simulink model "speed_modelo_motor_frenado"  (R2022b)
settings: Solver=VariableStepAuto  StartTime=0.0  StopTime=10  FixedStep=0.01  MaxStep=0.00005  RelTol=1e-3
values from neighbouring files (symbols this model uses):
  airgap_drag = [8 13 18 23]    [datos_modelo.mat]
  Force_drag = [-0.0263599613947 43.4567385798 79.8814932025 112.890713456 143.193346103 171.145741633 196.959308063 220.848934943 -0.0285293042528 24.6775545387 45.2474492116 63.9699604043 ... (32 elements, 8x4)]    [datos_modelo.mat]
  frecuencia = (3:3:48)    [carga_datos_motor_simple.m]    (also in datos_modelo.mat = [3 6 9 12 15 18 21 24 27 30 33 36 ... (16 elements, 1x16)])
  frecuencia_freno = -48:3:-3    [carga_datos_frenado_v3.m]    (also in carga_datos_frenado_v4.m; datos_modelo.mat = [-48 -45 -42 -39 -36 -33 -30 -27 -24 -21 -18 -15 ... (16 ele)
  FuerzaX_acel = []    [carga_datos_motor_simple.m]    (also in datos_modelo.mat = [0.156686825585 1.1015935563 2.01038201102 2.86930542934 3.6)
  FuerzaX_freno = []    [carga_datos_frenado_v3.m]    (also in datos_modelo.mat = [153.020892613 -180.239809195 -245.613894698 -262.756397176 )
  FuerzaY_acel = []    [carga_datos_motor_simple.m]    (also in datos_modelo.mat = [16.7719587108 16.6669307493 16.4360183454 16.0997979621 15.)
  Ipeak = (10:10:100)    [carga_datos_fuerza_laterales.m]    (also in carga_datos_motor_simple.m; datos_modelo.mat = [10 20 30 40 50 60 70 80 90 100])
  L = [0.00288301128086 0.00287460594326 0.00286413458194 0.00286292567045 0.00283652697085 0.00271657977235 0.0024764202896 0.0021234760901 0.00287319201871 0.00287259972172 0.0028679034407 0.0028580918991 ... (1408 elements, 8x11x16)]    [datos_modelo.mat]
  mass = 200    [datos_modelo.mat]
  p1 = 1.3    [datos_modelo.mat]
  p2 = 8.4    [datos_modelo.mat]
  pole_length = 0.114    [datos_modelo.mat]
  r = 0.384    [datos_modelo.mat]
  slip = (1:-0.1:0)    [carga_datos_motor_simple.m]    (also in datos_modelo.mat = [0 0.1 0.2 0.3 0.4 0.5 0.6 0.7 0.8 0.9 1])
  vel_drag = [0 5 10 15 20 25 30 35]    [datos_modelo.mat]
  vel_motor_freno = vel_motor_freno*3.6    [carga_datos_frenado_v3.m]    (also in datos_modelo.mat = [4.9248 9.8496 14.7744 19.6992 24.624 29.5488 34.4736 39.398)
libraries: slpidlib x2, eePowerMeasurement x1
settings Model: Creator=mique  LastModifiedBy=mique
settings SolverCC: ZeroCrossAlgorithm=Adaptive
settings DebuggingCC: IgnoredZcDiagnostic=none

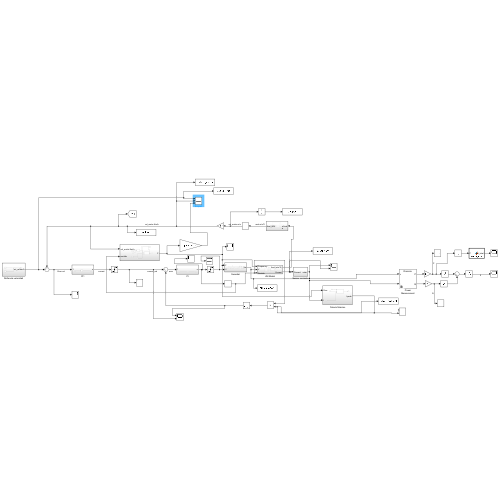
[thumbnail: Simulink's stored preview of the top-level diagram]
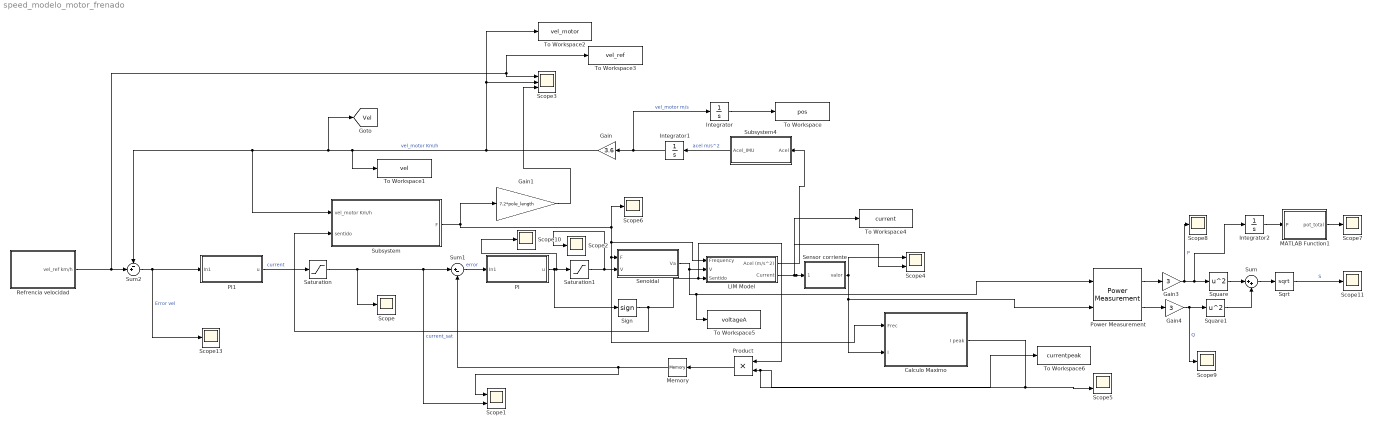
== system speed_modelo_motor_frenado ==
  Calculo Maximo : Subsystem
  Gain : Gain  Gain=3.6
  Gain1 : Gain  Gain=7.2*pole_length
  Gain3 : Gain  Gain=3
  Gain4 : Gain  Gain=3
  Integrator : Integrator
  Integrator1 : Integrator
  Integrator2 : Integrator
  LIM Model : Subsystem
  MATLAB Function1 : MATLAB Function  TreatAsAtomicUnit=on
  Memory : Memory
  PI : Subsystem
  PI1 : Subsystem
  Power Measurement : eePowerMeasurement/Power Measurement  LabelModeActiveChoice=Discrete  F=8  K=[0 1 2 3 4 5 6 7 8 9 10 11]  Ts=0.0002
  Product : Product
  Refrencia velocidad : Subsystem
  Saturation : Saturate  UpperLimit=100  LowerLimit=-100
  Saturation1 : Saturate  UpperLimit=200  LowerLimit=-200
  Scope{,2,6..11,13} (9 alike) : Scope
  Scope1 : Scope  NumInputPorts=2
  Scope3 : Scope  NumInputPorts=3
  Scope4 : Scope  NumInputPorts=2
  Scope5 : Scope  NumInputPorts=2
  Senoidal : Subsystem
  Sensor corriente : Subsystem
  Sign : Signum
  Sqrt : Sqrt
  Square : Math  Operator=square
  Square1 : Math  Operator=square
  Subsystem : Subsystem
  Subsystem4 : Subsystem
  Sum : Sum  Inputs=|++
  Sum1 : Sum  Inputs=|+-
  Sum2 : Sum  Inputs=-+|
  To Workspace : ToWorkspace  VariableName=pos  SampleTime=-1
  To Workspace1 : ToWorkspace  VariableName=vel  SampleTime=-1
  To Workspace2 : ToWorkspace  VariableName=vel_motor  SampleTime=-1
  To Workspace3 : ToWorkspace  VariableName=vel_ref  SampleTime=-1
  To Workspace4 : ToWorkspace  VariableName=current  SampleTime=-1
  To Workspace5 : ToWorkspace  VariableName=voltageA  SaveFormat=Timeseries  SampleTime=-1
  To Workspace6 : ToWorkspace  VariableName=currentpeak  SampleTime=-1
  tag scope: Vel=global
  wires:
  Integrator1/1 -> Integrator/1, Gain/1  "vel_motor m/s"
  Gain/1 -> To Workspace2/1, Scope3/2, To Workspace1/1, [Vel], Subsystem/1(vel_motor Km/h), Sum2/1  "vel_motor Km/h"
  LIM Model/1(Acel (m/s^2)) -> Subsystem4/1(Acel)
  Integrator/1 -> To Workspace/1
  Sum1/1 -> PI/1(In1)  "error"
  Sum2/1 -> PI1/1(In1), Scope13/1  "Error vel"
  Refrencia velocidad/1(vel_ref km/h) -> To Workspace3/1, Scope3/1, Sum2/2
  PI1/1(u) -> Saturation/1  "current"
  Gain1/1 -> Scope3/3
  Saturation/1 -> Scope/1, Scope1/2, Sum1/1  "current_sat"
  Subsystem4/1(Acel_IMU) -> Integrator1/1  "acel m/s^2"
  Senoidal/1(Va) -> To Workspace5/1, Power Measurement/1, LIM Model/2("V ")
  Power Measurement/1 -> Gain3/1
  Gain3/1 -> Integrator2/1, Square/1, Scope8/1  "P"
  Power Measurement/2 -> Gain4/1
  Gain4/1 -> Scope9/1, Square1/1  "Q"
  Square/1 -> Sum/1
  Square1/1 -> Sum/2
  Sum/1 -> Sqrt/1
  Sqrt/1 -> Scope11/1  "S"
  Sign/1 -> Subsystem/2(sentido), Product/1, LIM Model/3(Sentido)
  Product/1 -> Memory/1
  Memory/1 -> Scope1/1, Sum1/2
  Sensor corriente/1(valor) -> Scope4/1, Calculo Maximo/2(I), Power Measurement/2
  PI/1(u) -> Sign/1, Scope10/1, Saturation1/1
  Saturation1/1 -> Scope2/1, Senoidal/2(V)
  Integrator2/1 -> MATLAB Function1/1(P)
  MATLAB Function1/1(pot_total) -> Scope7/1
  Subsystem/1(F) -> Gain1/1, Scope6/1, Calculo Maximo/1(Frec), Senoidal/1(F), LIM Model/1(Frequency)
  Calculo Maximo/1(I peak) -> To Workspace6/1, Product/2, Scope5/2
  LIM Model/2(Current) -> Scope4/2, To Workspace4/1, Sensor corriente/1(Current)

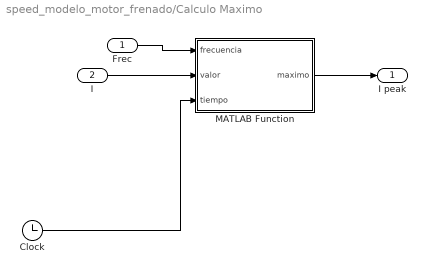
== system speed_modelo_motor_frenado/Calculo Maximo ==
  Frec : Inport
  I : Inport  Port=2
  Clock : Clock
  MATLAB Function : MATLAB Function  TreatAsAtomicUnit=on
  I peak : Outport
  wires:
  Frec/1 -> MATLAB Function/1(frecuencia)
  I/1 -> MATLAB Function/2(valor)
  MATLAB Function/1(maximo) -> I peak/1
  Clock/1 -> MATLAB Function/3(tiempo)

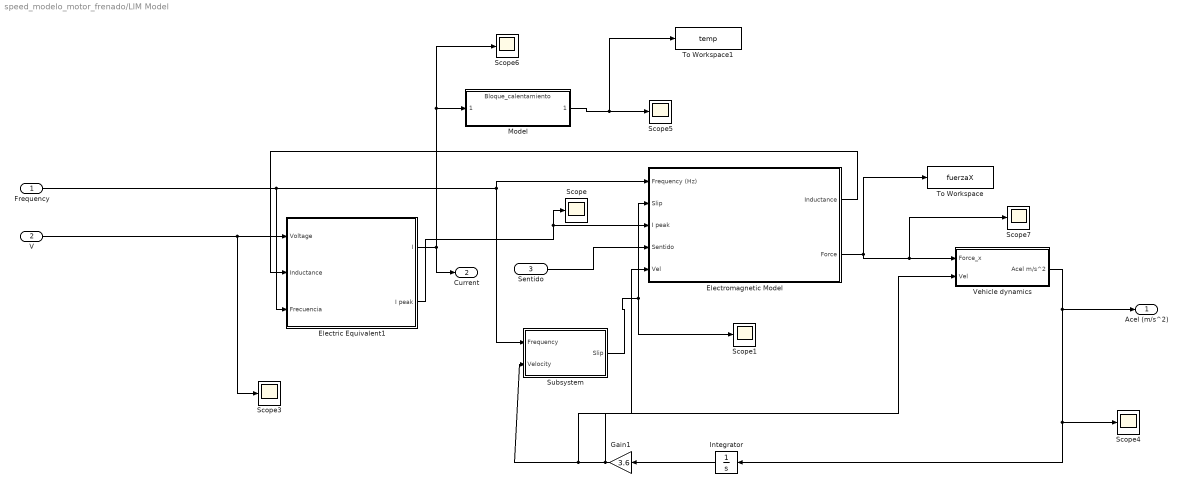
== system speed_modelo_motor_frenado/LIM Model ==
  Frequency : Inport
  "V " : Inport  Port=2
  Sentido : Inport  Port=3
  Electric Equivalent1 : Subsystem
  Electromagnetic Model : Subsystem
  Gain1 : Gain  Gain=3.6
  Integrator : Integrator
  Model : ModelReference  ModelNameDialog=Bloque_calentamiento.slx  SimulationMode=Normal  ModelReferenceVersion=3.8
  Scope{,1,3..7} (7 alike) : Scope
  Subsystem : Subsystem
  To Workspace : ToWorkspace  VariableName=fuerzaX  SampleTime=-1
  To Workspace1 : ToWorkspace  VariableName=temp  SampleTime=-1
  Vehicle dynamics : Subsystem
  Acel (m/s^2) : Outport
  Current : Outport  Port=2
  wires:
  Vehicle dynamics/1(Acel m/s^2) -> Integrator/1, Scope4/1, Acel (m/s^2)/1
  Electric Equivalent1/2(I peak) -> Scope/1, Electromagnetic Model/3(I peak)
  Electromagnetic Model/1(Inductance) -> Electric Equivalent1/2(Inductance)
  Frequency/1 -> Electric Equivalent1/3(Frecuencia), Subsystem/1(Frequency), Electromagnetic Model/1(Frequency (Hz))
  Integrator/1 -> Gain1/1
  "V "/1 -> Scope3/1, Electric Equivalent1/1(Voltage)
  Model/1 -> To Workspace1/1, Scope5/1
  Electric Equivalent1/1("I ") -> Current/1, Scope6/1, Model/1
  Sentido/1 -> Electromagnetic Model/4(Sentido)
  Subsystem/1(Slip) -> Scope1/1, Electromagnetic Model/2(Slip)
  Gain1/1 -> Vehicle dynamics/2(Vel), Electromagnetic Model/5(Vel), Subsystem/2(Velocity)
  Electromagnetic Model/2(Force) -> To Workspace/1, Scope7/1, Vehicle dynamics/1(Force_x)

== system speed_modelo_motor_frenado/PI ==
  note: Parametros obtenidos con el PID tuner
  In1 : Inport
  Discrete PID Controller1 : slpidlib/PID Controller  Controller=PI  Form=Parallel  TimeDomain=Discrete-time  UseExternalTs=off  SampleTime=0.0002  IntegratorMethod=Forward Euler  FilterMethod=Forward Euler  ControllerParametersSource=internal  P=0.3  I=5  UseKiTs=off  D=0.5  N=10  UseFilter=on  TunerSelectOption=Transfer Function Based (PID Tuner App)  InitialConditionSource=internal  InitialConditionForIntegrator=0  InitialConditionForFilter=0  DifferentiatorICPrevScaledInput=0  ExternalReset=none  TrackingMode=off  Kt=1  LimitOutput=off  SatLimitsSource=internal  UpperSaturationLimit=100  LowerSaturationLimit=-inf  LinearizeAsGain=off  AntiWindupMode=back-calculation  Kb=1  LimitIntegrator=off  UpperIntegratorSaturationLimit=15  LowerIntegratorSaturationLimit=-15  POutMin=[]  POutMax=[]  IOutMin=[]  IOutMax=[]  DOutMin=[]  DOutMax=[]  NOutMin=[]  NOutMax=[]  SumOutMin=[]  SumOutMax=[]  SaturationOutMin=[]  SaturationOutMax=[]  PParamMin=[]  PParamMax=[]  IParamMin=[]  IParamMax=[]  DParamMin=[]  DParamMax=[]  NParamMin=[]  NParamMax=[]  KbParamMin=[]  KbParamMax=[]  KtParamMin=[]  KtParamMax=[]  KbOutMin=[]  KbOutMax=[]  KtOutMin=[]  KtOutMax=[]  IntegratorOutMin=[]  IntegratorOutMax=[]  FilterOutMin=[]  FilterOutMax=[]  SumI1OutMin=[]  SumI1OutMax=[]  SumI2OutMin=[]  SumI2OutMax=[]  SumI3OutMin=[]  SumI3OutMax=[]  SumI4OutMin=[]  SumI4OutMax=[]  SumDOutMin=[]  SumDOutMax=[]  DifferentiatorOutMin=[]  DifferentiatorOutMax=[]  FilterDiffOutCoefMin=[]  FilterDiffOutCoefMax=[]  ReciprocalOutMin=[]  ReciprocalOutMax=[]  SumDenOutMin=[]  SumDenOutMax=[]  SumNumOutMin=[]  SumNumOutMax=[]  DivideOutMin=[]  DivideOutMax=[]  UdiffTsProdOutMin=[]  UdiffTsProdOutMax=[]  NTsProdOutMin=[]  NTsProdOutMax=[]  UintegralTsProdOutMin=[]  UintegralTsProdOutMax=[]  UngainTsProdOutMin=[]  UngainTsProdOutMax=[]  ClampingZeroOutDataTypeStr=Inherit: Inherit via back propagation  ClampingZeroOutMin=[]  ClampingZeroOutMax=[]  FilterDenConstantOutDataTypeStr=Inherit: Inherit via back propagation  FilterDenConstantOutMin=[]  FilterDenConstantOutMax=[]  PCopyOutDataTypeStr=Inherit: Inherit via back propagation  PCopyOutMin=[]  PCopyOutMax=[]  NCopyOutDataTypeStr=Inherit: Inherit via back propagation  NCopyOutMin=[]  NCopyOutMax=[]  IntegratorContinuousStateAttributes=''  IntegratorStateMustResolveToSignalObject=off  IntegratorRTWStateStorageClass=Auto  FilterContinuousStateAttributes=''  FilterStateMustResolveToSignalObject=off  FilterRTWStateStorageClass=Auto  ParallelPVariant=InternalParameters  IdealPVariant=Disabled  IVariant=InternalParameters  DVariant=Disabled  IntegratorVariant=Discrete  SatVariant=Disabled  AWVariant=Passthrough  PCopyVariant=Disabled  TRVariant=Disabled  FdbkBlocksVariant=Forward  IdealPFdbkVariant=Disabled  SatFdbkVariant=Disabled  DerivativeFilterVariant=Disabled  NVariant=Disabled  NCopyVariant=Disabled_SignalSpec  FilterICVariant=Disabled  IntegratorICVariant=InternalICs  ExternalResetVariant=Disabled  TRSumVariant=Passthrough  SumFdbkVariant=Disabled  SumVariant=Sum_PI  TsampFilterVariant=InternalTs  TsampNgainVariant=Passthrough  TsampIntegralVariant=Passthrough  ExternalSaturationOutDataTypeStr=Inherit: Same as second input
      settings: LibrarySourceBlock=simulink/Discrete/Discrete PID Controller
  u : Outport
  wires:
  In1/1 -> Discrete PID Controller1/1
  Discrete PID Controller1/1 -> u/1

== system speed_modelo_motor_frenado/PI1 ==
  note: Parametros obtenidos con el PID tuner
  In1 : Inport
  Discrete PID Controller1 : slpidlib/PID Controller  Controller=PI  Form=Parallel  TimeDomain=Discrete-time  UseExternalTs=off  SampleTime=0.001  IntegratorMethod=Forward Euler  FilterMethod=Forward Euler  ControllerParametersSource=internal  P=300  I=25  UseKiTs=off  D=0.2  N=10  UseFilter=on  TunerSelectOption=Transfer Function Based (PID Tuner App)  InitialConditionSource=internal  InitialConditionForIntegrator=0  InitialConditionForFilter=0  DifferentiatorICPrevScaledInput=0  ExternalReset=none  TrackingMode=off  Kt=1  LimitOutput=off  SatLimitsSource=internal  UpperSaturationLimit=100  LowerSaturationLimit=-100  LinearizeAsGain=off  AntiWindupMode=clamping  Kb=0.1  LimitIntegrator=on  UpperIntegratorSaturationLimit=15  LowerIntegratorSaturationLimit=-15  POutMin=[]  POutMax=[]  IOutMin=[]  IOutMax=[]  DOutMin=[]  DOutMax=[]  NOutMin=[]  NOutMax=[]  SumOutMin=[]  SumOutMax=[]  SaturationOutMin=[]  SaturationOutMax=[]  PParamMin=[]  PParamMax=[]  IParamMin=[]  IParamMax=[]  DParamMin=[]  DParamMax=[]  NParamMin=[]  NParamMax=[]  KbParamMin=[]  KbParamMax=[]  KtParamMin=[]  KtParamMax=[]  KbOutMin=[]  KbOutMax=[]  KtOutMin=[]  KtOutMax=[]  IntegratorOutMin=[]  IntegratorOutMax=[]  FilterOutMin=[]  FilterOutMax=[]  SumI1OutMin=[]  SumI1OutMax=[]  SumI2OutMin=[]  SumI2OutMax=[]  SumI3OutMin=[]  SumI3OutMax=[]  SumI4OutMin=[]  SumI4OutMax=[]  SumDOutMin=[]  SumDOutMax=[]  DifferentiatorOutMin=[]  DifferentiatorOutMax=[]  FilterDiffOutCoefMin=[]  FilterDiffOutCoefMax=[]  ReciprocalOutMin=[]  ReciprocalOutMax=[]  SumDenOutMin=[]  SumDenOutMax=[]  SumNumOutMin=[]  SumNumOutMax=[]  DivideOutMin=[]  DivideOutMax=[]  UdiffTsProdOutMin=[]  UdiffTsProdOutMax=[]  NTsProdOutMin=[]  NTsProdOutMax=[]  UintegralTsProdOutMin=[]  UintegralTsProdOutMax=[]  UngainTsProdOutMin=[]  UngainTsProdOutMax=[]  ClampingZeroOutDataTypeStr=Inherit: Inherit via back propagation  ClampingZeroOutMin=[]  ClampingZeroOutMax=[]  FilterDenConstantOutDataTypeStr=Inherit: Inherit via back propagation  FilterDenConstantOutMin=[]  FilterDenConstantOutMax=[]  PCopyOutDataTypeStr=Inherit: Inherit via back propagation  PCopyOutMin=[]  PCopyOutMax=[]  NCopyOutDataTypeStr=Inherit: Inherit via back propagation  NCopyOutMin=[]  NCopyOutMax=[]  IntegratorContinuousStateAttributes=''  IntegratorStateMustResolveToSignalObject=off  IntegratorRTWStateStorageClass=Auto  FilterContinuousStateAttributes=''  FilterStateMustResolveToSignalObject=off  FilterRTWStateStorageClass=Auto  ParallelPVariant=InternalParameters  IdealPVariant=Disabled  IVariant=InternalParameters  DVariant=Disabled  IntegratorVariant=Discrete  SatVariant=Disabled  AWVariant=Passthrough  PCopyVariant=Disabled  TRVariant=Disabled  FdbkBlocksVariant=Forward  IdealPFdbkVariant=Disabled  SatFdbkVariant=Disabled  DerivativeFilterVariant=Disabled  NVariant=Disabled  NCopyVariant=Disabled_SignalSpec  FilterICVariant=Disabled  IntegratorICVariant=InternalICs  ExternalResetVariant=Disabled  TRSumVariant=Passthrough  SumFdbkVariant=Disabled  SumVariant=Sum_PI  TsampFilterVariant=InternalTs  TsampNgainVariant=Passthrough  TsampIntegralVariant=Passthrough  ExternalSaturationOutDataTypeStr=Inherit: Same as second input
      settings: LibrarySourceBlock=simulink/Discrete/Discrete PID Controller
  u : Outport
  wires:
  Discrete PID Controller1/1 -> u/1
  In1/1 -> Discrete PID Controller1/1

== system speed_modelo_motor_frenado/Refrencia velocidad ==
  Step : Step  Time=4  After=35  SampleTime=0
  Step1 : Step  Time=5.90  After=-35  SampleTime=0
  Sum : Sum  Inputs=|++
  vel_ref km/h : Outport
  wires:
  Step/1 -> Sum/1
  Step1/1 -> Sum/2
  Sum/1 -> vel_ref km/h/1

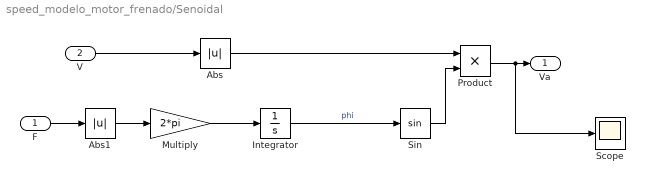
== system speed_modelo_motor_frenado/Senoidal ==
  F : Inport
  V : Inport  Port=2
  Abs : Abs  SaturateOnIntegerOverflow=off
  Abs1 : Abs  SaturateOnIntegerOverflow=off
  Integrator : Integrator  WrapState=on  WrappedStateUpperValue=2*pi  WrappedStateLowerValue=0
  Multiply : Gain  Gain=2*pi
  Product : Product
  Scope : Scope
  Sin : Trigonometry
  Va : Outport
  wires:
  Integrator/1 -> Sin/1  "phi"
  Sin/1 -> Product/2
  Product/1 -> Scope/1, Va/1
  F/1 -> Abs1/1
  Multiply/1 -> Integrator/1
  V/1 -> Abs/1
  Abs/1 -> Product/1
  Abs1/1 -> Multiply/1

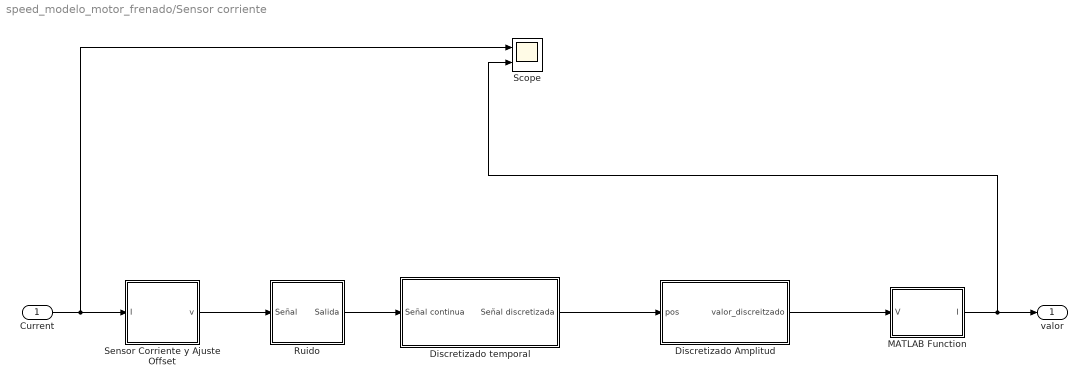
== system speed_modelo_motor_frenado/Sensor corriente ==
  Current : Inport
  Discretizado Amplitud : Subsystem  mask{Num_Val=4069, Max=4, Min=1}
      mask prompts: Num_Val "Numero de valores distintos"; Max "Maximo valor"; Min "Minimo valor"
  Discretizado temporal : Subsystem  mask{Tiempo_Discretizado=0.0002}
      mask prompts: Tiempo_Discretizado "Tiempo de discretizacion (s)"
      mask DialogControl DescGroupVar Prompt: Discretiza una señal mediante un ZOH con un tiempo definido
  MATLAB Function : MATLAB Function  TreatAsAtomicUnit=on
  Ruido : Subsystem  mask{M=0, V=0.00001, f=50}
      mask prompts: M "Media"; V "Varianza"; f "Frecuencia (Hz)"
      mask init:
      | T=1/f;
      mask DialogControl DescGroupVar Prompt: Añadidor de Ruido
      mask DialogControl DescTextVar Prompt: Añade un ruido blanco Gausiano con los siguientes valores:
  Scope : Scope  NumInputPorts=2
  Sensor Corriente y Ajuste Offset : Subsystem  mask{offset=0.0001, max=off}
      mask prompts: max "Offset positivo"
      mask init:
      | if(max==true)
      |         offset=abs(offset);
      | 
      |     else
      |         offset=-offset;
      |     end
  valor : Outport
  wires:
  Discretizado Amplitud/1(valor_discreitzado) -> MATLAB Function/1(V)
  Discretizado temporal/1(Señal discretizada) -> Discretizado Amplitud/1(pos)
  Sensor Corriente y Ajuste Offset/1(v) -> Ruido/1(Señal)
  Ruido/1(Salida) -> Discretizado temporal/1(Señal continua)
  Current/1 -> Scope/1, Sensor Corriente y Ajuste Offset/1(I)
  MATLAB Function/1(I) -> Scope/2, valor/1

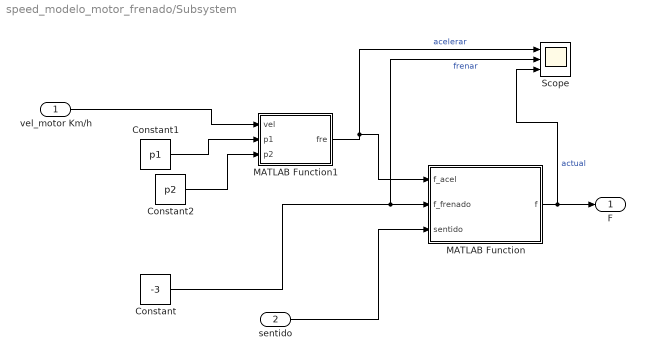
== system speed_modelo_motor_frenado/Subsystem ==
  vel_motor Km/h : Inport
  sentido : Inport  Port=2
  Constant : Constant  Value=-3
  Constant1 : Constant  Value=p1
  Constant2 : Constant  Value=p2
  MATLAB Function : MATLAB Function  TreatAsAtomicUnit=on
  MATLAB Function1 : MATLAB Function  TreatAsAtomicUnit=on
  Scope : Scope  NumInputPorts=3
  F : Outport
  wires:
  vel_motor Km/h/1 -> MATLAB Function1/1(vel)
  sentido/1 -> MATLAB Function/3(sentido)
  MATLAB Function1/1(fre) -> Scope/1, MATLAB Function/1(f_acel)  "acelerar"
  MATLAB Function/1(f) -> Scope/3, F/1  "actual"
  Constant1/1 -> MATLAB Function1/2(p1)
  Constant2/1 -> MATLAB Function1/3(p2)
  Constant/1 -> Scope/2, MATLAB Function/2(f_frenado)  "frenar"

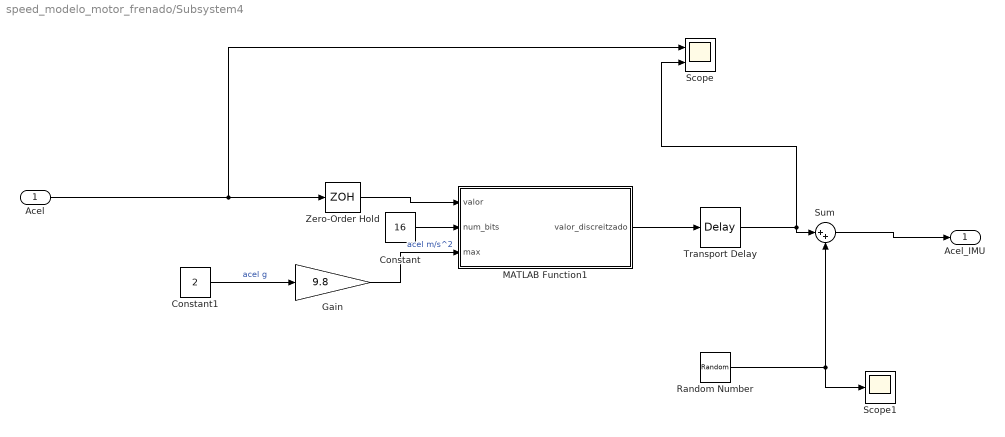
== system speed_modelo_motor_frenado/Subsystem4 ==
  Acel : Inport
  Constant : Constant  Value=16
  Constant1 : Constant  Value=2
  Gain : Gain  Gain=9.8
  MATLAB Function1 : MATLAB Function  TreatAsAtomicUnit=on
  Random Number : RandomNumber  Variance=0.1  SampleTime=0.001
  Scope : Scope  NumInputPorts=2
  Scope1 : Scope
  Sum : Sum  Inputs=|++
  Transport Delay : TransportDelay  DelayTime=0.001
  Zero-Order Hold : ZeroOrderHold  SampleTime=0.001
  Acel_IMU : Outport
  wires:
  MATLAB Function1/1(valor_discreitzado) -> Transport Delay/1
  Zero-Order Hold/1 -> MATLAB Function1/1(valor)
  Constant1/1 -> Gain/1  "acel g"
  Constant/1 -> MATLAB Function1/2(num_bits)
  Gain/1 -> MATLAB Function1/3(max)  "acel m/s^2"
  Transport Delay/1 -> Sum/1, Scope/2
  Acel/1 -> Scope/1, Zero-Order Hold/1
  Sum/1 -> Acel_IMU/1
  Random Number/1 -> Scope1/1, Sum/2

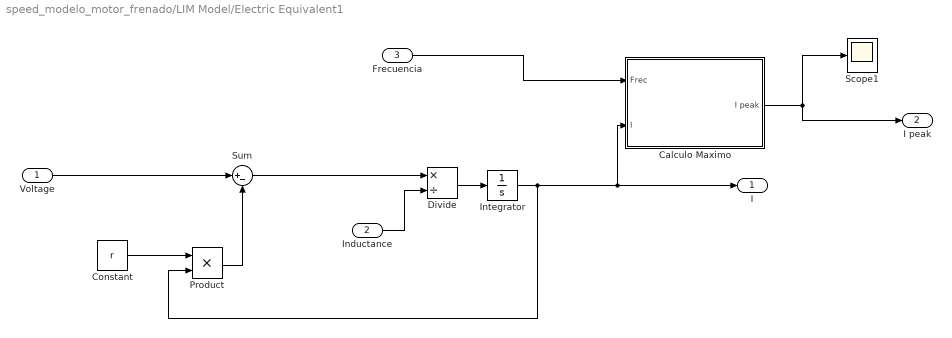
== system speed_modelo_motor_frenado/LIM Model/Electric Equivalent1 ==
  Voltage : Inport
  Inductance : Inport  Port=2
  Frecuencia : Inport  Port=3
  Calculo Maximo : Subsystem
  Constant : Constant  Value=r
  Divide : Product  Inputs=*/
  Integrator : Integrator
  Product : Product
  Scope1 : Scope
  Sum : Sum  Inputs=|+-
  "I " : Outport
  I peak : Outport  Port=2
  wires:
  Voltage/1 -> Sum/1
  Integrator/1 -> Calculo Maximo/2(I), "I "/1, Product/2
  Constant/1 -> Product/1
  Product/1 -> Sum/2
  Divide/1 -> Integrator/1
  Sum/1 -> Divide/1
  Inductance/1 -> Divide/2
  Calculo Maximo/1(I peak) -> I peak/1, Scope1/1
  Frecuencia/1 -> Calculo Maximo/1(Frec)

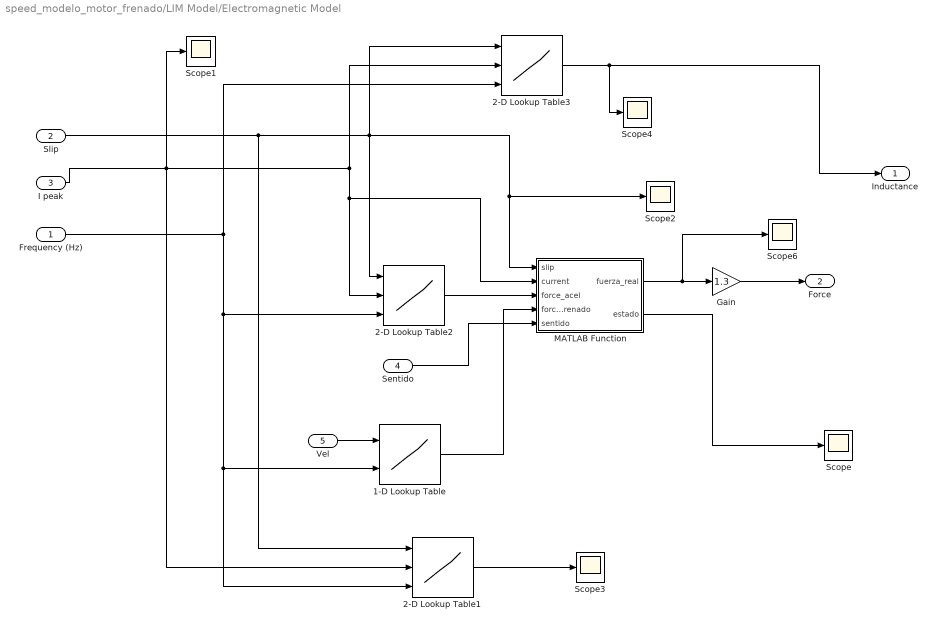
== system speed_modelo_motor_frenado/LIM Model/Electromagnetic Model ==
  Frequency (Hz) : Inport
  Slip : Inport  Port=2
  I peak : Inport  Port=3
  Sentido : Inport  Port=4
  Vel : Inport  Port=5
  1-D Lookup Table : Lookup_n-D  BreakpointsForDimension1=vel_motor_freno  BreakpointsForDimension2=frecuencia_freno  Table=FuerzaX_freno  InternalRulePriority=Speed  RndMeth=Simplest
      settings: InputPortMap=u0,u1
  2-D Lookup Table1 : Lookup_n-D  NumberOfTableDimensions=3  BreakpointsForDimension1=slip  BreakpointsForDimension2=Ipeak  BreakpointsForDimension3=frecuencia  Table=FuerzaY_acel  InterpMethod=Nearest  InternalRulePriority=Speed  RndMeth=Simplest
      settings: InputPortMap=u0,u1,u2
  2-D Lookup Table2 : Lookup_n-D  NumberOfTableDimensions=3  BreakpointsForDimension1=slip  BreakpointsForDimension2=Ipeak  BreakpointsForDimension3=frecuencia  Table=FuerzaX_acel  InternalRulePriority=Speed  RndMeth=Simplest
      settings: InputPortMap=u0,u1,u2
  2-D Lookup Table3 : Lookup_n-D  NumberOfTableDimensions=3  BreakpointsForDimension1=Ipeak(2:(end-1))  BreakpointsForDimension2=slip  BreakpointsForDimension3=frecuencia  Table=L  InterpMethod=Nearest  InternalRulePriority=Speed  RndMeth=Simplest
      settings: InputPortMap=u0,u1,u2
  Gain : Gain  Gain=1.3
  MATLAB Function : MATLAB Function  TreatAsAtomicUnit=on
  Scope{,1..4,6} (6 alike) : Scope
  Inductance : Outport
  Force : Outport  Port=2
  wires:
  2-D Lookup Table3/1 -> Scope4/1, Inductance/1
  Frequency (Hz)/1 -> 1-D Lookup Table/2, 2-D Lookup Table1/3, 2-D Lookup Table2/3, 2-D Lookup Table3/3
  I peak/1 -> 2-D Lookup Table1/2, MATLAB Function/2(current), 2-D Lookup Table2/2, 2-D Lookup Table3/2, Scope1/1
  Slip/1 -> 2-D Lookup Table1/1, Scope2/1, MATLAB Function/1(slip), 2-D Lookup Table2/1, 2-D Lookup Table3/1
  2-D Lookup Table2/1 -> MATLAB Function/3(force_acel)
  2-D Lookup Table1/1 -> Scope3/1
  Sentido/1 -> MATLAB Function/5(sentido)
  MATLAB Function/2(estado) -> Scope/1
  MATLAB Function/1(fuerza_real) -> Scope6/1, Gain/1
  Gain/1 -> Force/1
  1-D Lookup Table/1 -> MATLAB Function/4(force_frenado)
  Vel/1 -> 1-D Lookup Table/1

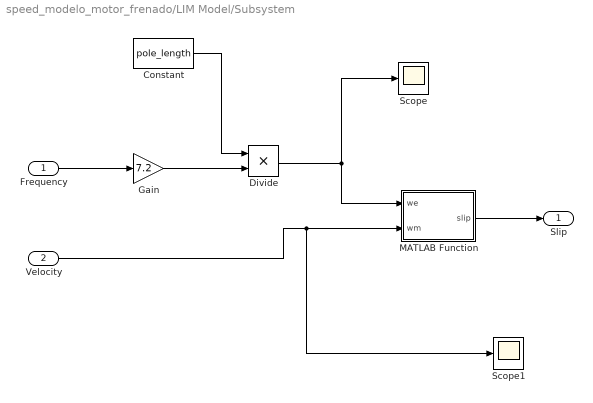
== system speed_modelo_motor_frenado/LIM Model/Subsystem ==
  Frequency : Inport
  Velocity : Inport  Port=2
  Constant : Constant  Value=pole_length
  Divide : Product  Inputs=**
  Gain : Gain  Gain=7.2
  MATLAB Function : MATLAB Function  TreatAsAtomicUnit=on
  Scope : Scope
  Scope1 : Scope
  Slip : Outport
  wires:
  Frequency/1 -> Gain/1
  MATLAB Function/1(slip) -> Slip/1
  Gain/1 -> Divide/2
  Constant/1 -> Divide/1
  Divide/1 -> Scope/1, MATLAB Function/1(we)
  Velocity/1 -> Scope1/1, MATLAB Function/2(wm)

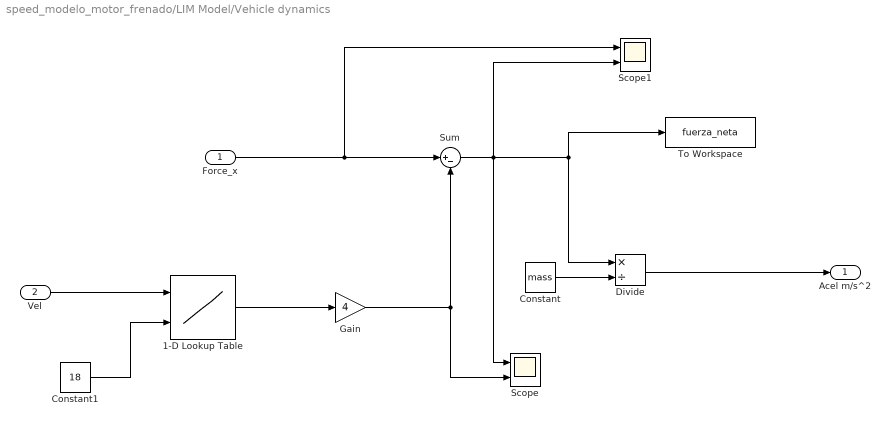
== system speed_modelo_motor_frenado/LIM Model/Vehicle dynamics ==
  Force_x : Inport
  Vel : Inport  Port=2
  1-D Lookup Table : Lookup_n-D  BreakpointsForDimension1=vel_drag  BreakpointsForDimension2=airgap_drag  Table=Force_drag  InternalRulePriority=Speed  RndMeth=Simplest
      settings: InputPortMap=u0,u1
  Constant : Constant  Value=mass
  Constant1 : Constant  Value=18
  Divide : Product  Inputs=*/
  Gain : Gain  Gain=4
  Scope : Scope  NumInputPorts=2
  Scope1 : Scope  NumInputPorts=2
  Sum : Sum  Inputs=|+-
  To Workspace : ToWorkspace  VariableName=fuerza_neta  SampleTime=-1
  Acel m/s^2 : Outport
  wires:
  Divide/1 -> Acel m/s^2/1
  Constant/1 -> Divide/2
  Force_x/1 -> Sum/1, Scope1/1
  Sum/1 -> To Workspace/1, Divide/1, Scope1/2, Scope/1
  Constant1/1 -> 1-D Lookup Table/2
  1-D Lookup Table/1 -> Gain/1
  Gain/1 -> Scope/2, Sum/2
  Vel/1 -> 1-D Lookup Table/1

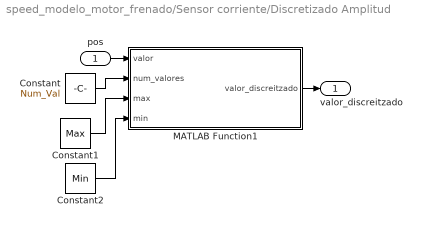
== system speed_modelo_motor_frenado/Sensor corriente/Discretizado Amplitud ==
  pos : Inport
  Constant : Constant  Value=Num_Val
  Constant1 : Constant  Value=Max
  Constant2 : Constant  Value=Min
  MATLAB Function1 : MATLAB Function  TreatAsAtomicUnit=on
  valor_discreitzado : Outport
  wires:
  pos/1 -> MATLAB Function1/1(valor)
  Constant2/1 -> MATLAB Function1/4(min)
  Constant/1 -> MATLAB Function1/2(num_valores)
  Constant1/1 -> MATLAB Function1/3(max)
  MATLAB Function1/1(valor_discreitzado) -> valor_discreitzado/1

== system speed_modelo_motor_frenado/Sensor corriente/Discretizado temporal ==
  Señal continua : Inport
  Zero-Order Hold : ZeroOrderHold  SampleTime=Tiempo_Discretizado
  Señal discretizada : Outport
  wires:
  Zero-Order Hold/1 -> Señal discretizada/1
  Señal continua/1 -> Zero-Order Hold/1

== system speed_modelo_motor_frenado/Sensor corriente/Ruido ==
  Señal : Inport
  Ruido : RandomNumber  Mean=M  Variance=V  Seed=10  SampleTime=T
  Sum : Sum  Inputs=|++
  Salida : Outport
  wires:
  Sum/1 -> Salida/1
  Ruido/1 -> Sum/1
  Señal/1 -> Sum/2

== system speed_modelo_motor_frenado/Sensor corriente/Sensor Corriente y Ajuste Offset ==
  I : Inport
  Constant : Constant  Value=offset
  Sensor : MATLAB Function  TreatAsAtomicUnit=on
  v : Outport
  wires:
  I/1 -> Sensor/1(I)
  Constant/1 -> Sensor/2(offset)
  Sensor/1(V_o) -> v/1

== system speed_modelo_motor_frenado/LIM Model/Electric Equivalent1/Calculo Maximo ==
  Frec : Inport
  I : Inport  Port=2
  Clock : Clock
  MATLAB Function : MATLAB Function  TreatAsAtomicUnit=on
  I peak : Outport
  wires:
  Frec/1 -> MATLAB Function/1(frecuencia)
  I/1 -> MATLAB Function/2(valor)
  MATLAB Function/1(maximo) -> I peak/1
  Clock/1 -> MATLAB Function/3(tiempo)

== matlab function speed_modelo_motor_frenado/Calculo Maximo/MATLAB Function ==
  settings: updateMethod=DISCRETE
  data: frecuencia input; maximo output; valor input; tiempo input
function maximo = fcn(frecuencia,valor,tiempo)

   persistent antiguo_maximo
    if isempty(antiguo_maximo)
       antiguo_maximo=0;
    end
    persistent t_maximo
    if isempty(t_maximo)
       t_maximo=0;
    end

periodo=1/abs(frecuencia);


if abs(valor)>=antiguo_maximo
    maximo=abs(valor);
    antiguo_maximo=abs(valor);
    t_maximo=tiempo;
else
    maximo=antiguo_maximo;
    if tiempo>t_maximo+periodo
        maximo=abs(valor);
        antiguo_maximo=abs(valor);
        t_maximo=tiempo;
    end
end

== matlab function speed_modelo_motor_frenado/LIM Model/Electromagnetic Model/MATLAB Function ==
  data: slip input; fuerza_real output; current input; force_acel input; force_frenado input; sentido input; estado output
function [fuerza_real,estado]= fcn(slip,current,force_acel,force_frenado,sentido)

if sentido>=0
    force=force_acel;
    estado=1;
else
    force=force_frenado;
    estado=2;
end

if slip == 0 || current<4 && current>-4

    fuerza_real=0;
    estado=3;

else
    fuerza_real=force;
    estado=4;
end

== matlab function speed_modelo_motor_frenado/Sensor corriente/Discretizado Amplitud/MATLAB Function1 ==
  data: valor input; valor_discreitzado output; num_valores input; max input; min input
function valor_discreitzado  = fcn(valor,num_valores,max,min)

if(valor>max)
    valor_discreitzado=max;
    return
end
if(valor<min)
    valor_discreitzado=min;
    return
end


valor_escalon=(max-min)/(num_valores-1);


i=min;
 while(i<max)
    if(i+valor_escalon/2>valor)
        valor_discreitzado=i;
        return
    end
    i=i+valor_escalon;
end



      valor_discreitzado=max;
end

== matlab function speed_modelo_motor_frenado/LIM Model/Electric Equivalent1/Calculo Maximo/MATLAB Function ==
  settings: updateMethod=DISCRETE
  data: frecuencia input; maximo output; valor input; tiempo input
function maximo = fcn(frecuencia,valor,tiempo)

   persistent antiguo_maximo
    if isempty(antiguo_maximo)
       antiguo_maximo=0;
    end
    persistent t_maximo
    if isempty(t_maximo)
       t_maximo=0;
    end

periodo=1/abs(frecuencia);


if abs(valor)>=antiguo_maximo
    maximo=abs(valor);
    antiguo_maximo=abs(valor);
    t_maximo=tiempo;
else
    maximo=antiguo_maximo;
    if tiempo>t_maximo+periodo
        maximo=abs(valor);
        antiguo_maximo=abs(valor);
        t_maximo=tiempo;
    end
end

== matlab function speed_modelo_motor_frenado/LIM Model/Subsystem/MATLAB Function ==
  data: we input; slip output; wm input
function slip = fcn(we,wm)

slip = (we-wm)/we;

== matlab function speed_modelo_motor_frenado/Subsystem/MATLAB Function1 ==
  data: vel input; fre output; p1 input; p2 input
function fre = fcn(vel,p1,p2)

fre=p2+p1*vel;

== matlab function speed_modelo_motor_frenado/Subsystem/MATLAB Function ==
  data: f_acel input; f output; f_frenado input; sentido input
function f= fcn(f_acel,f_frenado,sentido)

if sentido>=0
    f=f_acel;

else
    f=f_frenado;

end

== matlab function speed_modelo_motor_frenado/MATLAB Function1 ==
  data: P input; pot_total output
function pot_total = efecto_total(P)

pot_total=0;
for k=1:max(size(P))
    pot_total=pot_total+P(k);
end

== matlab function speed_modelo_motor_frenado/Sensor corriente/MATLAB Function ==
  data: V input; I output
function I = fcn(V)

I=(V-2.5)/0.005;

== matlab function speed_modelo_motor_frenado/Subsystem4/MATLAB Function1 ==
  data: valor input; valor_discreitzado output; num_bits input; max input
function valor_discreitzado  = fcn(valor,num_bits,max)

min=-max;
num_valores=2^num_bits;
if(valor>max)
    valor_discreitzado=max;
    return
end
if(valor<min)
    valor_discreitzado=min;
    return
end


valor_escalon=(max-min)/(num_valores-1);


i=min;
 while(i<max)
    if(i+valor_escalon/2>valor)
        valor_discreitzado=i;
        return
    end
    i=i+valor_escalon;
end



      valor_discreitzado=max;
end

== matlab function speed_modelo_motor_frenado/Sensor corriente/Sensor Corriente y Ajuste Offset/Sensor ==
  data: I input; V_o output; offset input
function V_o = Sensor_L01Z300S05(I,offset)
Vcc=5;
if(I>300)
    I=300;
end
if(I<-300)
    I=-300;
end
V_ref=Vcc/2;
V_o=V_ref+0.005*I;

V_o=V_o+offset;

end
